simulink model "curiosity_i2c_pitch_roll"  (R2024b)
settings: Solver=FixedStepDiscrete  StartTime=0.0  StopTime=inf  FixedStep=1e-3  RelTol=1e-3  EnableMultiTasking=on
undefined symbols (not defined in the file): A0, ADC, D10, D7, D8, D9, DiscIntNeverNeededParam, Max, MaxPer, ms, NumBits1, NumBits2, P1, P58, P59, Pin, Resol, s, Timer, us
libraries: MCHP_Blockset x18, simulink x15, dspstat3 x1
(part 3 of 4)

== system curiosity_i2c_pitch_roll/Final_roll_pitch ==
  Roll_Accel : Inport
  Pitch_Accel : Inport  Port=2
  Roll_Gyro : Inport  Port=3
  Pitch_Gyro : Inport  Port=4
  Add1 : Sum
  Add2 : Sum
  HPF : Subsystem
  HPF1 : Subsystem
  LPF : Subsystem
  LPF1 : Subsystem
  Roll : Outport
  Pitch : Outport  Port=2
  wires:
  Add1/1 -> Pitch/1
  Roll_Accel/1 -> LPF/1("Rollin ")
  Roll_Gyro/1 -> HPF/1("Rollin ")
  LPF/1(Rollout) -> Add2/1
  HPF/1(Rollout) -> Add2/2
  Add2/1 -> Roll/1
  Pitch_Accel/1 -> LPF1/1(Pitchin)
  Pitch_Gyro/1 -> HPF1/1(Pitchin)
  LPF1/1(Pitchout) -> Add1/1
  HPF1/1(Pitchout) -> Add1/2

== system curiosity_i2c_pitch_roll/Gyro_bias_clculator ==
  Gx : Inport
  Gy : Inport  Port=2
  Gz : Inport  Port=3
  Enable : EnablePort
  Data Type Conversion3 : DataTypeConversion  Commented=on  OutDataTypeStr=single  SaturateOnIntegerOverflow=off  RndMeth=Floor
  Mean3 : dspstat3/Mean  Commented=on  run=on  InputProcessing=Columns as channels (frame based)  reset_popup=None  directionMode=Each column  dimension=1  roiEnable=off  roiType=Rectangles  roiPortion=Entire ROI  roiOutput=Individual statistics for each ROI  roiFlag=off  roundingMode=Floor  overflowMode=off  outputDataTypeStr=Inherit: Same as accumulator  outputMin=[]  outputMax=[]  outputLastDataTypeStr=Inherit: Same as accumulator
  manu_mean1 : Subsystem
  manu_mean2 : Subsystem
  manu_mean3 : Subsystem
  Gx_bias : Outport
  Gy_bias : Outport  Port=2
  Gz_bias : Outport  Port=3
  wires:
  Gx/1 -> manu_mean3/1(Ax)
  manu_mean3/1(Ax_bias1) -> Gx_bias/1
  Mean3/1 -> ?
  ? -> Data Type Conversion3/1
  Data Type Conversion3/1 -> Mean3/1
  manu_mean1/1(Ax_bias1) -> Gy_bias/1
  Gy/1 -> manu_mean1/1(Ax)
  Gz/1 -> manu_mean2/1(Ax)
  manu_mean2/1(Ax_bias1) -> Gz_bias/1

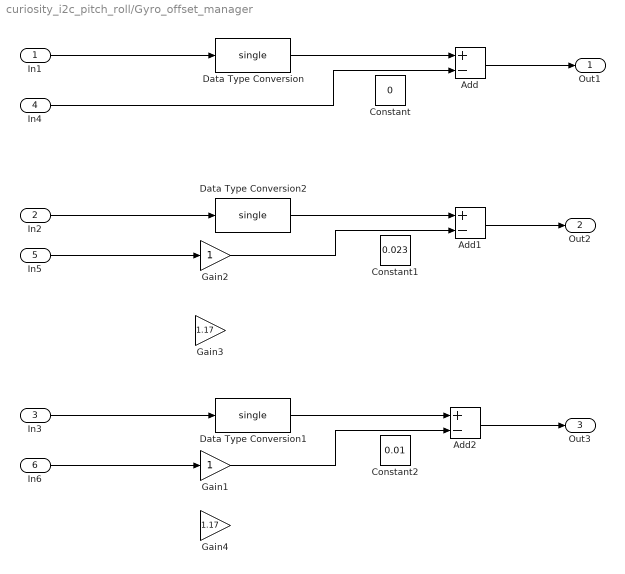
== system curiosity_i2c_pitch_roll/Gyro_offset_manager ==
  In1 : Inport
  In2 : Inport  Port=2
  In3 : Inport  Port=3
  In4 : Inport  Port=4
  In5 : Inport  Port=5
  In6 : Inport  Port=6
  Add : Sum  Inputs=+-
  Add1 : Sum  Inputs=+-
  Add2 : Sum  Inputs=+-
  Constant : Constant  Value=0  SampleTime=0.005
  Constant1 : Constant  Value=0.023  SampleTime=0.005
  Constant2 : Constant  Value=0.01  SampleTime=0.005
  Data Type Conversion : DataTypeConversion  OutDataTypeStr=single  SaturateOnIntegerOverflow=off  RndMeth=Floor
  Data Type Conversion1 : DataTypeConversion  OutDataTypeStr=single  SaturateOnIntegerOverflow=off  RndMeth=Floor
  Data Type Conversion2 : DataTypeConversion  OutDataTypeStr=single  SaturateOnIntegerOverflow=off  RndMeth=Floor
  Gain1 : Gain
  Gain2 : Gain
  Gain3 : Gain  Gain=1.17
  Gain4 : Gain  Gain=1.17
  Out1 : Outport
  Out2 : Outport  Port=2
  Out3 : Outport  Port=3
  wires:
  In3/1 -> Data Type Conversion1/1
  In1/1 -> Data Type Conversion/1
  In2/1 -> Data Type Conversion2/1
  Data Type Conversion/1 -> Add/1
  Data Type Conversion2/1 -> Add1/1
  Data Type Conversion1/1 -> Add2/1
  Add/1 -> Out1/1
  Add1/1 -> Out2/1
  Add2/1 -> Out3/1
  In5/1 -> Gain2/1
  In6/1 -> Gain1/1
  In4/1 -> Add/2
  Gain1/1 -> Add2/2
  Gain2/1 -> Add1/2

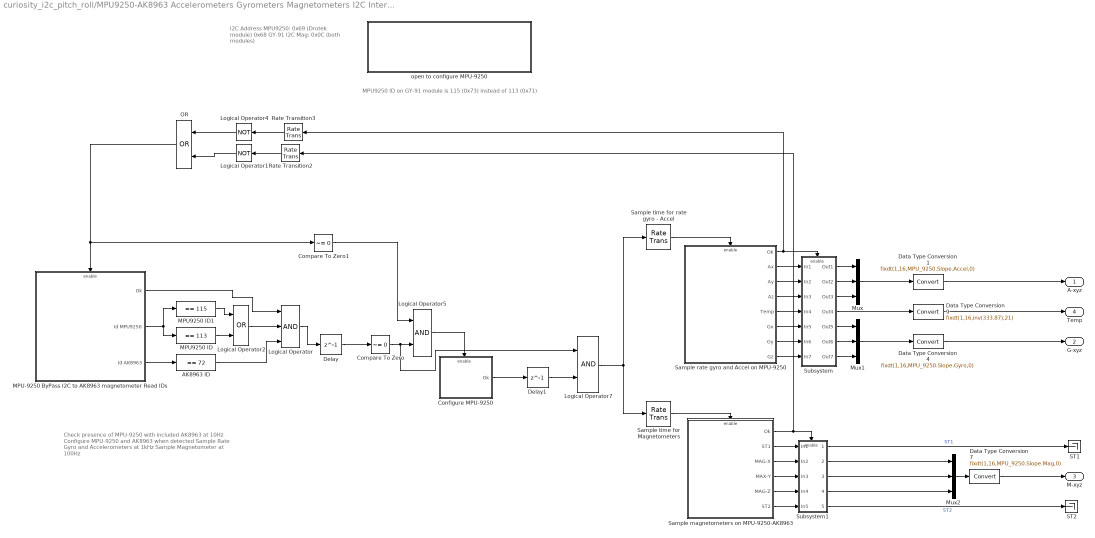
== system curiosity_i2c_pitch_roll/MPU9250-AK8963 Accelerometers Gyrometers Magnetometers I2C Interface ==
  note: I2C Address MPU9250:
      | 0x69 (Drotek module)
      | 0x68 GY-91
      |
      | I2C Mag:
      | 0x0C (both modules)
  note: MPU9250 ID on GY-91 module is 115 (0x73) instead of 113 (0x71)
  note: Check presence of MPU-9250 with included AK8963 at 10Hz
      | Configure MPU-9250 and AK8963 when detected
      | Sample Rate Gyro and Accelerometers at 1kHz
      | Sample Magnetometer at 100Hz
  AK8963 ID : simulink/Logic and Bit Operations/Compare To Constant  relop===  const=72  OutDataTypeStr=boolean
  Compare To Zero : simulink/Logic and Bit Operations/Compare To Zero  relop=~=  OutDataTypeStr=boolean
  Compare To Zero1 : simulink/Logic and Bit Operations/Compare To Zero  relop=~=  OutDataTypeStr=boolean
  Configure MPU-9250 : Subsystem  Priority=-90
  Data Type Conversion1 : DataTypeConversion  OutDataTypeStr=fixdt(1,16,MPU_9250.Slope.Accel,0)  ConvertRealWorld=Stored Integer (SI)  SaturateOnIntegerOverflow=off  RndMeth=Floor
  Data Type Conversion4 : DataTypeConversion  OutDataTypeStr=fixdt(1,16,MPU_9250.Slope.Gyro,0)  ConvertRealWorld=Stored Integer (SI)  SaturateOnIntegerOverflow=off  RndMeth=Floor
  Data Type Conversion7 : DataTypeConversion  OutDataTypeStr=fixdt(1,16,MPU_9250.Slope.Mag,0)  ConvertRealWorld=Stored Integer (SI)  SaturateOnIntegerOverflow=off  RndMeth=Floor
  Data Type Conversion9 : DataTypeConversion  OutDataTypeStr=fixdt(1,16,inv(333.87),21)  ConvertRealWorld=Stored Integer (SI)  SaturateOnIntegerOverflow=off  RndMeth=Floor
  Delay : Delay  DelayLength=1  InitialCondition=0
  Delay1 : Delay  DelayLength=1  InitialCondition=0
  Logical Operator : Logic  Inputs=3  AllPortsSameDT=off  OutDataTypeStr=boolean
  Logical Operator1 : Logic  Operator=NOT  AllPortsSameDT=off  OutDataTypeStr=boolean
  Logical Operator2 : Logic  Operator=OR  AllPortsSameDT=off  OutDataTypeStr=boolean
  Logical Operator4 : Logic  Operator=NOT  AllPortsSameDT=off  OutDataTypeStr=boolean
  Logical Operator5 : Logic  AllPortsSameDT=off  OutDataTypeStr=boolean
  Logical Operator7 : Logic  AllPortsSameDT=off  OutDataTypeStr=boolean
  MPU-9250 ByPass I2C to AK8963 magnetometer Read IDs : Subsystem
  MPU9250 ID : simulink/Logic and Bit Operations/Compare To Constant  relop===  const=113  OutDataTypeStr=boolean
  MPU9250 ID1 : simulink/Logic and Bit Operations/Compare To Constant  relop===  const=115  OutDataTypeStr=boolean
  Mux : Mux  Inputs=3
  Mux1 : Mux  Inputs=3
  Mux2 : Mux  Inputs=3
  OR : Logic  Operator=OR  AllPortsSameDT=off  OutDataTypeStr=boolean
  Rate Transition2 : RateTransition  Deterministic=off
  Rate Transition3 : RateTransition  Deterministic=off
  ST1 : Terminator
  ST2 : Terminator
  Sample magnetometers on MPU-9250-AK8963 : Subsystem
  Sample rate gyro and Accel on MPU-9250 : Subsystem  Priority=0
  Sample time for rate gyro - Accel : RateTransition  Deterministic=off  OutPortSampleTime=.005
  Sample time for Magnetometers : RateTransition  Deterministic=off  OutPortSampleTime=[.01 0.003]
  Subsystem : Subsystem
  Subsystem1 : Subsystem
  open to configure MPU-9250 : Subsystem  Priority=-500  LoadFcn=|  mask{ADDR=0x68 with AD0 Logic Low, GYRO_FS_SEL=250 deg/s, GYRO_DLPFCFG=92Hz - 3.9ms delay (Fs=1kHz), ACCEL_FS_SEL=4g, ACCEL_DLPFCFG=44.8 Hz - 4.88ms delay (Fs=1kHz), evalin_variableName=MPU_9250, evalin_ws=MPU_9250.Slope.Gyro=MCHP_Fun.Hex2num('3F21740AFA84AD89');MPU_9250.Slope.Accel=MCHP_Fun.Hex2num('3F539EB851EB851F');MPU_9250.Slope.Mag=0.15;MPU_9250.ADDR=104;MPU_9250.Config=2;MPU_9250.Gyro_Config=0;MPU_9250.Accel_Config=8;MPU_9250.Accel_Config2=3;}
      | txt = get_param(gcbh,'evalin_ws');
      | evalin('base',txt);
      mask prompts: ADDR "MPU9250 I2C 7 bit address"; GYRO_FS_SEL "Gyro Full Scale Select"; GYRO_DLPFCFG "Gyro Bandwidth"; ACCEL_FS_SEL "Accel Full Scale Select"; ACCEL_DLPFCFG "Accel Bandwidth"; evalin_variableName "evalin workSpace variable:"
      mask init:
      | MPU_9250.Slope.Gyro = sscanf(GYRO_FS_SEL,'%d')*2^-15*pi/180; % in radian/s
      | MPU_9250.Slope.Accel = sscanf(ACCEL_FS_SEL,'%d')*2^-15 * 9.81; % in m/s^2
      | MPU_9250.Slope.Mag = 0.15; % 0.15uT/LSB
      | 
      | switch ADDR
      |     case '0x68 with AD0 Logic Low'
      |         G_ADDR = hex2dec('68');
      |     case '0x69 with AD0 Logic High'
      |         G_ADDR = hex2dec('69');
      | end
      | 
      | switch GYRO_FS_SEL
      |     case '250 deg/s'
      |     	G_FS_SEL = 0;
      | 	case '500 deg/s'
      | 		G_FS_SEL = 1;
      | 	case '1000 deg/s'
      | 		G_FS_SEL = 2;
      | 	case '2000 deg/s'
      | 		G_FS_SEL = 3;
      | end
      | 
      | switch GYRO_DLPFCFG
      | 	case '8800Hz - 0.064ms delay (Fs=32kHz)'
      | 		FCHOICE = 0;
      | 		G_DLPF_CFG = 0; % don't care
      | 	case '3600Hz - 0.11ms delay (Fs=32kHz)'
      | 		FCHOICE = 1;
      | 		G_DLPF_CFG = 0; % don't care
      | 	case '3600Hz - 0.17ms delay (Fs=8kHz)'
      | 		FCHOICE = 3;
      | 		G_DLPF_CFG = 7;
      | 	case '250Hz - 0.97ms delay (Fs=8kHz)'
      | 		FCHOICE = 3;
      | 		G_DLPF_CFG = 0;
      | 	case '184Hz - 2.9ms delay (Fs=1kHz)'
      | 		FCHOICE = 3;
      | 		G_DLPF_CFG = 1;
      | 	case '92Hz - 3.9ms delay (Fs=1kHz)'
      | 		FCHOICE = 3;
      | 		G_DLPF_CFG = 2;
      | 	case '41Hz - 5.9ms delay (Fs=1kHz)'
      | 		FCHOICE = 3;
      | 		G_DLPF_CFG = 3;
      | 	case '20Hz - 9.9ms delay (Fs=1kHz)'
      | 		FCHOICE = 3;
      | 		G_DLPF_CFG = 4;
      | 	case '10Hz - 17.85ms delay (Fs=1kHz)'
      | 		FCHOICE = 3;
      | 		G_DLPF_CFG = 5;
      | 	case '5Hz - 33.48ms delay (Fs=1kHz)'
      | 		FCHOICE = 3;
      | 		G_DLPF_CFG = 6;      
      | end
      | 
      | switch ACCEL_FS_SEL
      | 	case '2g'
      | 		A_FS_SEL = 0;        
      | 	case '4g'
      | 		A_FS_SEL = 1;        
      | 	case '8g'
      | 		A_FS_SEL = 2;        
      | 	case '16g'
      | 		A_FS_SEL = 3;        
      | end
      | 
      | switch ACCEL_DLPFCFG
      | 	case '1046 Hz - 0.0503ms delay (Fs=4kHz)'
      | 		A_FCHOICE_B = 0;
      | 		A_DLPF_CFG = 0; % don't care
      | 	case '420.0 Hz - 1.38ms delay (Fs=1kHz)'
      | 		A_FCHOICE_B = 1;
      | 		A_DLPF_CFG = 7;
      | 	case '218.1 Hz - 1.88ms delay (Fs=1kHz)'
      | 		A_FCHOICE_B = 1;
      | 		A_DLPF_CFG = 1;
      | 	case '99.0 Hz - 2.88ms delay (Fs=1kHz)'
      | 		A_FCHOICE_B = 1;
      | 		A_DLPF_CFG = 2;
      | 	case '44.8 Hz - 4.88ms delay (Fs=1kHz)'
      | 		A_FCHOICE_B = 1;
      | 		A_DLPF_CFG = 3;
      | 	case '21.2 Hz - 8.87ms delay (Fs=1kHz)'
      | 		A_FCHOICE_B = 1;
      | 		A_DLPF_CFG = 4;
      | 	case '10.2 Hz - 16.83ms delay (Fs=1kHz)'
      | 		A_FCHOICE_B = 1;
      | 		A_DLPF_CFG = 5;
      | 	case '5.05 Hz - 32.48ms delay (Fs=1kHz)'
      | 		A_FCHOICE_B = 1;
      | 		A_DLPF_CFG = 6;
      | end
      | 
      | 
      | MPU_9250.ADDR = G_ADDR;
      | MPU_9250.Config = G_DLPF_CFG;
      | MPU_9250.Gyro_Config = G_FS_SEL * 2^3 + bitxor(FCHOICE,3);
      | MPU_9250.Accel_Config = A_FS_SEL * 2^3;
      | MPU_9250.Accel_Config2 = bitxor(A_FCHOICE_B,1)*2^2 + A_DLPF_CFG;
      | 
      | txt = MCHP_Fun.Struct2txt(MPU_9250,evalin_variableName);
      | set_param(gcbh,'evalin_ws',txt);
      | 
      | assignin('base',evalin_variableName,MPU_9250);
      | 
      | %mdlWks = get_param(bdroot,'ModelWorkspace');
      | %assignin(mdlWks,'MPU_9250',MPU_9250);
      mask TypeOptions ADDR: 0x68 with AD0 Logic Low | 0x69 with AD0 Logic High
      mask TypeOptions GYRO_FS_SEL: 250 deg/s | 500 deg/s | 1000 deg/s | 2000 deg/s
      mask TypeOptions GYRO_DLPFCFG: 8800Hz - 0.064ms delay (Fs=32kHz) | 3600Hz - 0.11ms delay (Fs=32kHz) | 3600Hz - 0.17ms delay (Fs=8kHz) | 250Hz - 0.97ms delay (Fs=8kHz) | 184Hz - 2.9ms delay (Fs=1kHz) | 92Hz - 3.9ms delay (Fs=1kHz) | 41Hz - 5.9ms delay (Fs=1kHz) | 20Hz - 9.9ms delay (Fs=1kHz) | 10Hz - 17.85ms delay (Fs=1kHz) | 5Hz - 33.48ms delay (Fs=1kHz)
      mask TypeOptions ACCEL_FS_SEL: 2g | 4g | 8g | 16g
      mask TypeOptions ACCEL_DLPFCFG: 1046 Hz - 0.0503ms delay (Fs=4kHz) | 420.0 Hz - 1.38ms delay (Fs=1kHz) | 218.1 Hz - 1.88ms delay (Fs=1kHz) | 99.0 Hz - 2.88ms delay (Fs=1kHz) | 44.8 Hz - 4.88ms delay (Fs=1kHz) | 21.2 Hz - 8.87ms delay (Fs=1kHz) | 10.2 Hz - 16.83ms delay (Fs=1kHz) | 5.05 Hz - 32.48ms delay (Fs=1kHz)
      mask Display: disp(['MPU-9250\n\nG: +-' GYRO_FS_SEL ' - ' GYRO_DLPFCFG '\nA: +-' ACCEL_FS_SEL ' - ' ACCEL_DLPFCFG '\nvariable --> ' evalin_variableName]);
  A-xyz : Outport  Unit=m/s^2  VectorParamsAs1DForOutWhenUnconnected=off
  G-xyz : Outport  Port=2  Unit=rad/s  VectorParamsAs1DForOutWhenUnconnected=off
  M-xyz : Outport  Port=3  Unit=µT  VectorParamsAs1DForOutWhenUnconnected=off
  Temp : Outport  Port=4  Unit=°C  VectorParamsAs1DForOutWhenUnconnected=off
  wires:
  Delay1/1 -> Logical Operator7/2
  MPU-9250 ByPass I2C to AK8963 magnetometer Read IDs/1(Ok) -> Logical Operator/1
  Logical Operator5/1 -> Configure MPU-9250/Enable
  Compare To Zero1/1 -> Logical Operator5/1
  Delay/1 -> Compare To Zero/1
  Compare To Zero/1 -> Logical Operator5/2, Logical Operator7/1
  OR/1 -> Compare To Zero1/1, MPU-9250 ByPass I2C to AK8963 magnetometer Read IDs/Enable
  Subsystem1/5(Out5) -> ST2/1  "ST2"
  Subsystem1/4(Out4) -> Mux2/3
  Subsystem1/3(Out3) -> Mux2/2
  Subsystem1/2(Out2) -> Mux2/1
  Subsystem1/1(Out1) -> ST1/1  "ST1"
  Sample magnetometers on MPU-9250-AK8963/6(ST2) -> Subsystem1/5(In5)
  Sample magnetometers on MPU-9250-AK8963/5(MAG-Z) -> Subsystem1/4(In4)
  Sample magnetometers on MPU-9250-AK8963/4(MAX-Y) -> Subsystem1/3(In3)
  Sample magnetometers on MPU-9250-AK8963/3(MAG-X) -> Subsystem1/2(In2)
  Sample magnetometers on MPU-9250-AK8963/2(ST1) -> Subsystem1/1(In1)
  Subsystem/7(Out7) -> Mux1/3
  Subsystem/6(Out6) -> Mux1/2
  Subsystem/5(Out5) -> Mux1/1
  Subsystem/4(Out4) -> Data Type Conversion9/1
  Subsystem/3(Out3) -> Mux/3
  Subsystem/2(Out2) -> Mux/2
  Subsystem/1(Out1) -> Mux/1
  Sample rate gyro and Accel on MPU-9250/8(Gz) -> Subsystem/7(In7)
  Sample rate gyro and Accel on MPU-9250/7(Gy) -> Subsystem/6(In6)
  Sample rate gyro and Accel on MPU-9250/6(Gx) -> Subsystem/5(In5)
  Sample rate gyro and Accel on MPU-9250/5(Temp) -> Subsystem/4(In4)
  Sample rate gyro and Accel on MPU-9250/4(Az) -> Subsystem/3(In3)
  Sample rate gyro and Accel on MPU-9250/3(Ay) -> Subsystem/2(In2)
  Sample rate gyro and Accel on MPU-9250/2(Ax) -> Subsystem/1(In1)
  Data Type Conversion4/1 -> G-xyz/1
  Data Type Conversion9/1 -> Temp/1
  Data Type Conversion1/1 -> A-xyz/1
  Logical Operator7/1 -> Sample time for rate gyro - Accel/1, Sample time for Magnetometers/1
  Configure MPU-9250/1(Ok) -> Delay1/1
  Logical Operator/1 -> Delay/1
  Sample time for Magnetometers/1 -> Sample magnetometers on MPU-9250-AK8963/Enable
  MPU9250 ID/1 -> Logical Operator2/2
  Sample time for rate gyro - Accel/1 -> Sample rate gyro and Accel on MPU-9250/Enable
  Logical Operator1/1 -> OR/2
  Logical Operator2/1 -> Logical Operator/2
  Mux2/1 -> Data Type Conversion7/1
  Logical Operator4/1 -> OR/1
  Rate Transition2/1 -> Logical Operator1/1
  MPU-9250 ByPass I2C to AK8963 magnetometer Read IDs/2(Id MPU9250) -> MPU9250 ID1/1, MPU9250 ID/1
  Data Type Conversion7/1 -> M-xyz/1
  MPU-9250 ByPass I2C to AK8963 magnetometer Read IDs/3("Id AK8963 ") -> AK8963 ID/1
  Mux/1 -> Data Type Conversion1/1
  Sample magnetometers on MPU-9250-AK8963/1(Ok) -> Rate Transition2/1, Subsystem1/Enable
  AK8963 ID/1 -> Logical Operator/3
  MPU9250 ID1/1 -> Logical Operator2/1
  Rate Transition3/1 -> Logical Operator4/1
  Sample rate gyro and Accel on MPU-9250/1(Ok) -> Subsystem/Enable, Rate Transition3/1
  Mux1/1 -> Data Type Conversion4/1

== system curiosity_i2c_pitch_roll/Roll_&_Pitch_Acel ==
  Ax : Inport
  Ay : Inport  Port=2
  Az : Inport  Port=3
  Add : Sum
  Ay1 : InportShadow  Port=2
  Az1 : InportShadow  Port=3
  Gain : Gain  Gain=-1
  Gain1 : Gain  Gain=57.29
  Gain2 : Gain  Gain=57.29
  Sqrt : Sqrt
  Square : Math  Operator=square
  Square1 : Math  Operator=square
  Trigonometric Function1 : Trigonometry  Operator=atan2  ApproximationMethod=Lookup  TableDataTypeStr=single
  Trigonometric Function2 : Trigonometry  Operator=atan2  ApproximationMethod=Lookup  TableDataTypeStr=single
  Roll_angle : Outport
  Pitch_angle : Outport  Port=2
  wires:
  Square1/1 -> Add/2
  Gain/1 -> Trigonometric Function2/1
  Sqrt/1 -> Trigonometric Function2/2
  Add/1 -> Sqrt/1
  Square/1 -> Add/1
  Ay/1 -> Trigonometric Function1/1
  Az/1 -> Trigonometric Function1/2
  Trigonometric Function1/1 -> Gain1/1
  Ax/1 -> Gain/1
  Ay1/1 -> Square/1
  Az1/1 -> Square1/1
  Trigonometric Function2/1 -> Gain2/1
  Gain1/1 -> Roll_angle/1
  Gain2/1 -> Pitch_angle/1

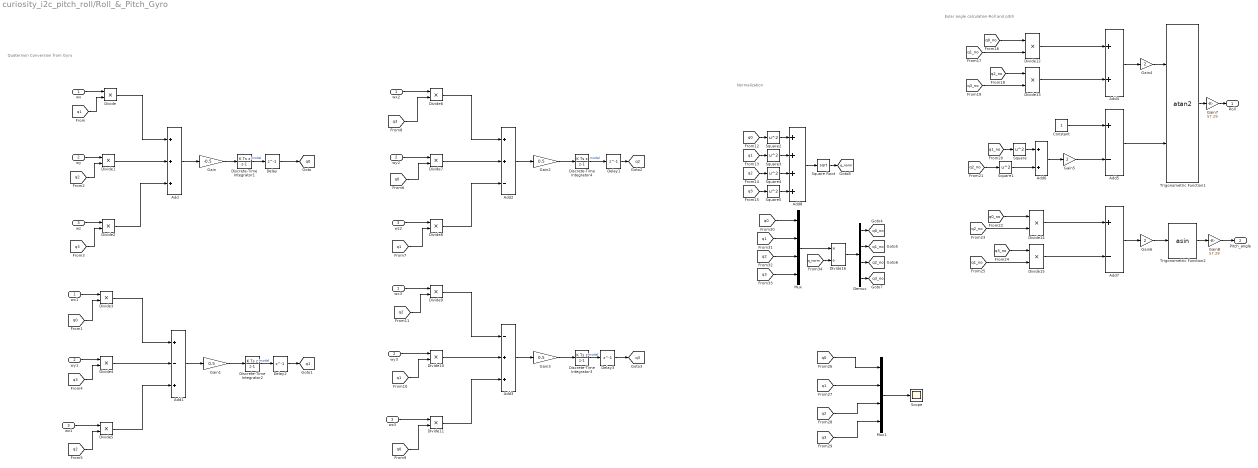
== system curiosity_i2c_pitch_roll/Roll_&_Pitch_Gyro ==
  note: Eular angle calculation-Roll and pitch
  note: Normalization
  note: Quaternion Conversion from Gyro
  wx : Inport
  wy : Inport  Port=2
  wz : Inport  Port=3
  Add : Sum  Inputs=+++
  Add1 : Sum  Inputs=+-+
  Add2 : Sum  Inputs=++-
  Add3 : Sum  Inputs=-++
  Add4 : Sum
  Add5 : Sum  Inputs=+-
  Add6 : Sum
  Add7 : Sum  Inputs=+-
  Add8 : Sum  Inputs=++++
  Constant : Constant  OutDataTypeStr=single  SampleTime=0.005
  Delay : Delay  DelayLength=1  InitialCondition=1  InputProcessing=Columns as channels (frame based)
  Delay1 : Delay  DelayLength=1  InputProcessing=Columns as channels (frame based)
  Delay2 : Delay  DelayLength=1  InputProcessing=Columns as channels (frame based)
  Delay3 : Delay  DelayLength=1  InputProcessing=Columns as channels (frame based)
  Demux : Demux
  Discrete-Time Integrator1 : DiscreteIntegrator  IntegratorMethod=Integration: Backward Euler  InitialCondition=1  SampleTime=-1  OutDataTypeStr=single  ICPrevOutput=DiscIntNeverNeededParam  ICPrevScaledInput=DiscIntNeverNeededParam
  Discrete-Time Integrator2 : DiscreteIntegrator  IntegratorMethod=Integration: Backward Euler  SampleTime=-1  OutDataTypeStr=single  ICPrevOutput=DiscIntNeverNeededParam  ICPrevScaledInput=DiscIntNeverNeededParam
  Discrete-Time Integrator3 : DiscreteIntegrator  IntegratorMethod=Integration: Backward Euler  SampleTime=-1  OutDataTypeStr=single  ICPrevOutput=DiscIntNeverNeededParam  ICPrevScaledInput=DiscIntNeverNeededParam
  Discrete-Time Integrator4 : DiscreteIntegrator  IntegratorMethod=Integration: Backward Euler  SampleTime=-1  OutDataTypeStr=single  ICPrevOutput=DiscIntNeverNeededParam  ICPrevScaledInput=DiscIntNeverNeededParam
  Divide{,1..15} (16 alike) : Product  Inputs=**
  Divide16 : Product  Inputs=*/
  Gain : Gain  Gain=-0.5
  Gain1 : Gain  Gain=0.5
  Gain2 : Gain  Gain=0.5
  Gain3 : Gain  Gain=0.5
  Gain4 : Gain  Gain=2
  Gain5 : Gain  Gain=2
  Gain6 : Gain  Gain=2
  Gain7 : Gain  Gain=57.29
  Gain8 : Gain  Gain=57.29
  Mux : Mux
  Mux1 : Mux
  Scope : Scope
  Square{,1..5} (6 alike) : Math  Operator=square
  Square Root : Sqrt
  Trigonometric Function1 : Trigonometry  Operator=atan2  ApproximationMethod=Lookup  TableDataTypeStr=single
  Trigonometric Function2 : Trigonometry  Operator=asin  ApproximationMethod=Lookup  TableDataTypeStr=single
  wx1 : InportShadow
  wx2 : InportShadow
  wx3 : InportShadow
  wy1 : InportShadow  Port=2
  wy2 : InportShadow  Port=2
  wy3 : InportShadow  Port=2
  wz1 : InportShadow  Port=3
  wz2 : InportShadow  Port=3
  wz3 : InportShadow  Port=3
  Roll : Outport
  Pitch_angle : Outport  Port=2
  tag scope: q0=global, q0_no=global, q1=global, q1_no=global, q2=global, q2_no=global, q3=global, q3_no=global, q_norm=global
  wires:
  [q0] -> Square2/1
  [q1] -> Square3/1
  [q2] -> Square4/1
  [q3] -> Square5/1
  Divide12/1 -> Add4/1
  [q1_no] -> Divide12/2
  [q2_no] -> Divide13/1
  Divide13/1 -> Add4/2
  [q3_no] -> Divide13/2
  Add4/1 -> Gain4/1
  Gain4/1 -> Trigonometric Function1/1
  Constant/1 -> Add5/1
  Gain5/1 -> Add5/2
  [q1_no] -> Square/1
  Add6/1 -> Gain5/1
  Square/1 -> Add6/1
  [q2_no] -> Square1/1
  Square1/1 -> Add6/2
  Add5/1 -> Trigonometric Function1/2
  [q1_no] -> Divide15/2
  Divide15/1 -> Add7/2
  [q3_no] -> Divide15/1
  [q2_no] -> Divide14/2
  [q0_no] -> Divide14/1
  Divide14/1 -> Add7/1
  Add7/1 -> Gain6/1
  Gain6/1 -> Trigonometric Function2/1
  Trigonometric Function2/1 -> Gain8/1
  [q0] -> Mux1/1
  Mux1/1 -> Scope/1
  [q1] -> Mux1/2
  [q2] -> Mux1/3
  [q3] -> Mux1/4
  Square2/1 -> Add8/1
  Square3/1 -> Add8/2
  Square4/1 -> Add8/3
  Square5/1 -> Add8/4
  Add8/1 -> Square Root/1
  Square Root/1 -> [q_norm]
  [q0] -> Mux/1
  [q1] -> Mux/2
  [q2] -> Mux/3
  [q3] -> Mux/4
  Mux/1 -> Divide16/1
  [q_norm] -> Divide16/2
  Divide16/1 -> Demux/1
  Demux/1 -> [q0_no]
  Demux/2 -> [q1_no]
  Demux/3 -> [q2_no]
  Demux/4 -> [q3_no]
  [q0_no] -> Divide12/1
  Divide4/1 -> Add1/2
  Add3/1 -> Gain3/1
  Add1/1 -> Gain1/1
  Divide9/1 -> Add3/1
  Discrete-Time Integrator1/1 -> Delay/1  "model"
  Divide11/1 -> Add3/3
  wz1/1 -> Divide5/1
  Delay2/1 -> [q1]
  wx/1 -> Divide/1
  Discrete-Time Integrator2/1 -> Delay2/1  "model"
  Divide8/1 -> Add2/3
  wx2/1 -> Divide6/1
  [q0] -> Divide11/2
  Gain/1 -> Discrete-Time Integrator1/1
  wx1/1 -> Divide3/1
  Divide/1 -> Add/1
  [q3] -> Divide4/2
  wz2/1 -> Divide8/1
  Discrete-Time Integrator3/1 -> Delay3/1  "model"
  wx3/1 -> Divide9/1
  Divide3/1 -> Add1/1
  [q3] -> Divide2/2
  Add2/1 -> Gain2/1
  Add/1 -> Gain/1
  Divide2/1 -> Add/3
  Discrete-Time Integrator4/1 -> Delay1/1  "model"
  [q2] -> Divide5/2
  Delay1/1 -> [q2]
  wz/1 -> Divide2/1
  wy/1 -> Divide1/1
  [q2] -> Divide9/2
  Divide7/1 -> Add2/2
  [q2] -> Divide1/2
  Gain2/1 -> Discrete-Time Integrator4/1
  [q0] -> Divide7/2
  Divide5/1 -> Add1/3
  wy3/1 -> Divide10/1
  Divide1/1 -> Add/2
  Gain3/1 -> Discrete-Time Integrator3/1
  Gain1/1 -> Discrete-Time Integrator2/1
  Divide10/1 -> Add3/2
  Divide6/1 -> Add2/1
  [q3] -> Divide6/2
  wy1/1 -> Divide4/1
  Delay/1 -> [q0]
  wy2/1 -> Divide7/1
  Delay3/1 -> [q3]
  [q1] -> Divide10/2
  [q1] -> Divide8/2
  [q0] -> Divide3/2
  wz3/1 -> Divide11/1
  [q1] -> Divide/2
  Trigonometric Function1/1 -> Gain7/1
  Gain7/1 -> Roll/1
  Gain8/1 -> Pitch_angle/1

== system curiosity_i2c_pitch_roll/Sine Wave Generator Use dsPIC A hardware sine fct ==
  In1 : Inport
  Bias : Bias  Bias=0.5  SaturateOnIntegerOverflow=off
  Cast3 : DataTypeConversion  OutDataTypeStr=single  SaturateOnIntegerOverflow=off  RndMeth=Floor
  Discrete-Time Integrator3 : DiscreteIntegrator  gainval=1  SampleTime=.01  OutDataTypeStr=fixdt(0,16,16)  RndMeth=Simplest  ICPrevOutput=DiscIntNeverNeededParam  ICPrevScaledInput=DiscIntNeverNeededParam
      settings: LockScale=on
  Gain : Gain  Gain=0.5
  Gain2 : Gain  Gain=2*pi
  Sin3 : Trigonometry  OutputSignalType=real
  Out1 : Outport
  wires:
  In1/1 -> Discrete-Time Integrator3/1
  Discrete-Time Integrator3/1 -> Cast3/1
  Bias/1 -> Out1/1
  Gain2/1 -> Sin3/1
  Sin3/1 -> Gain/1
  Cast3/1 -> Gain2/1
  Gain/1 -> Bias/1

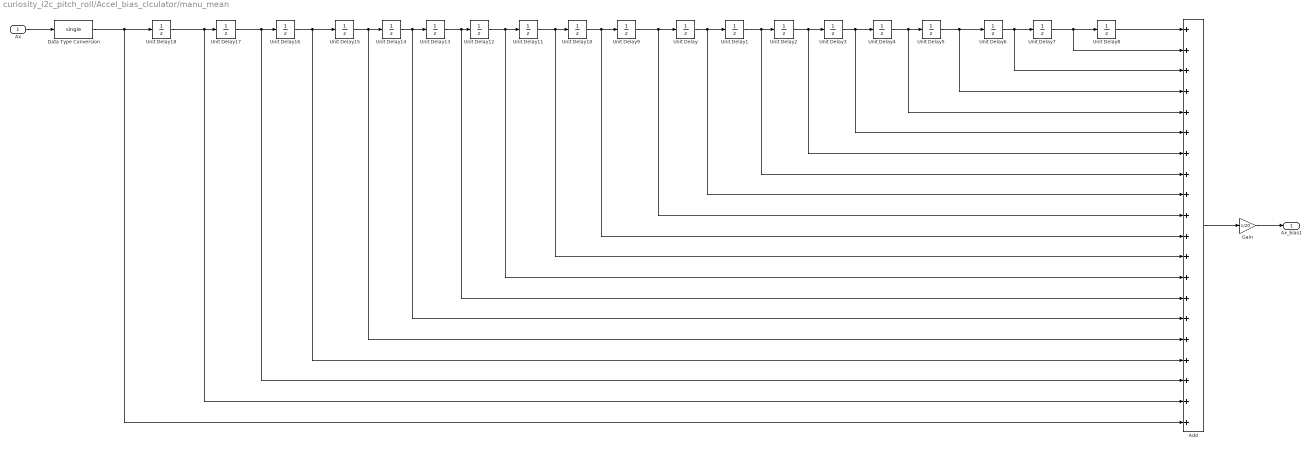
== system curiosity_i2c_pitch_roll/Accel_bias_clculator/manu_mean ==
  Ax : Inport
  Add : Sum  Inputs=++++++++++++++++++++
  Data Type Conversion : DataTypeConversion  OutDataTypeStr=single  SaturateOnIntegerOverflow=off  RndMeth=Floor
  Gain : Gain  Gain=1/20
  Unit Delay{,1..18} (19 alike) : UnitDelay  SampleTime=-1  HasFrameUpgradeWarning=on
  Ax_bias1 : Outport
  wires:
  Unit Delay2/1 -> Add/7, Unit Delay3/1
  Unit Delay1/1 -> Add/8, Unit Delay2/1
  Unit Delay/1 -> Add/9, Unit Delay1/1
  Unit Delay7/1 -> Add/2, Unit Delay8/1
  Unit Delay5/1 -> Add/4, Unit Delay6/1
  Unit Delay4/1 -> Add/5, Unit Delay5/1
  Unit Delay3/1 -> Add/6, Unit Delay4/1
  Unit Delay6/1 -> Add/3, Unit Delay7/1
  Data Type Conversion/1 -> Add/20, Unit Delay18/1
  Add/1 -> Gain/1
  Ax/1 -> Data Type Conversion/1
  Unit Delay8/1 -> Add/1
  Gain/1 -> Ax_bias1/1
  Unit Delay9/1 -> Add/10, Unit Delay/1
  Unit Delay10/1 -> Add/11, Unit Delay9/1
  Unit Delay11/1 -> Add/12, Unit Delay10/1
  Unit Delay12/1 -> Add/13, Unit Delay11/1
  Unit Delay13/1 -> Add/14, Unit Delay12/1
  Unit Delay14/1 -> Add/15, Unit Delay13/1
  Unit Delay15/1 -> Add/16, Unit Delay14/1
  Unit Delay16/1 -> Add/17, Unit Delay15/1
  Unit Delay17/1 -> Add/18, Unit Delay16/1
  Unit Delay18/1 -> Add/19, Unit Delay17/1

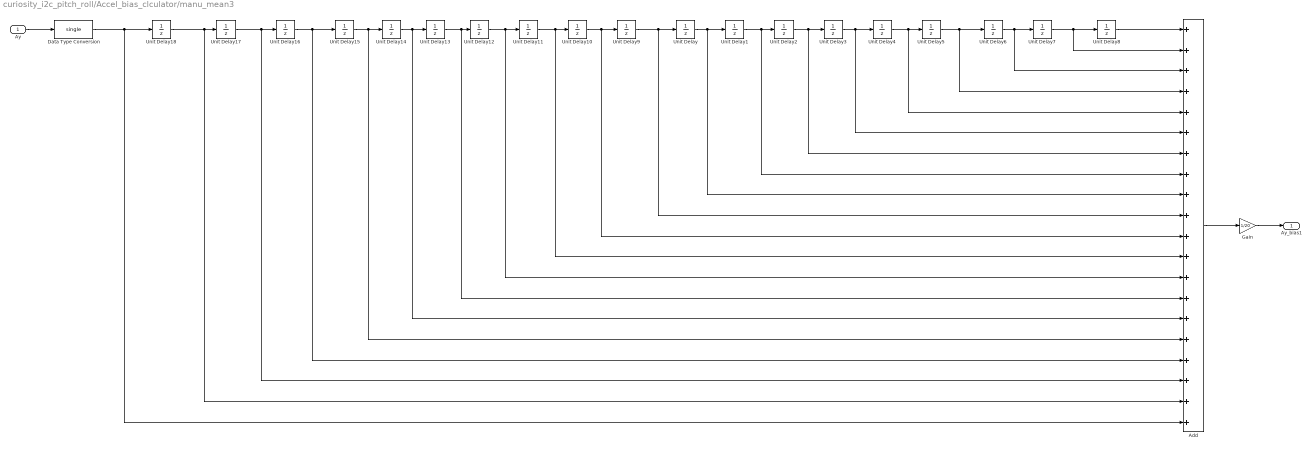
== system curiosity_i2c_pitch_roll/Accel_bias_clculator/manu_mean3 ==
  Ay : Inport
  Add : Sum  Inputs=++++++++++++++++++++
  Data Type Conversion : DataTypeConversion  OutDataTypeStr=single  SaturateOnIntegerOverflow=off  RndMeth=Floor
  Gain : Gain  Gain=1/20
  Unit Delay{,1..18} (19 alike) : UnitDelay  SampleTime=-1  HasFrameUpgradeWarning=on
  Ay_bias1 : Outport
  wires:
  Unit Delay18/1 -> Unit Delay17/1, Add/19
  Unit Delay17/1 -> Unit Delay16/1, Add/18
  Unit Delay16/1 -> Unit Delay15/1, Add/17
  Unit Delay15/1 -> Unit Delay14/1, Add/16
  Unit Delay14/1 -> Unit Delay13/1, Add/15
  Unit Delay13/1 -> Unit Delay12/1, Add/14
  Unit Delay12/1 -> Unit Delay11/1, Add/13
  Unit Delay11/1 -> Unit Delay10/1, Add/12
  Unit Delay10/1 -> Unit Delay9/1, Add/11
  Unit Delay9/1 -> Unit Delay/1, Add/10
  Gain/1 -> Ay_bias1/1
  Unit Delay8/1 -> Add/1
  Ay/1 -> Data Type Conversion/1
  Add/1 -> Gain/1
  Data Type Conversion/1 -> Unit Delay18/1, Add/20
  Unit Delay6/1 -> Unit Delay7/1, Add/3
  Unit Delay3/1 -> Unit Delay4/1, Add/6
  Unit Delay4/1 -> Unit Delay5/1, Add/5
  Unit Delay5/1 -> Unit Delay6/1, Add/4
  Unit Delay7/1 -> Unit Delay8/1, Add/2
  Unit Delay/1 -> Unit Delay1/1, Add/9
  Unit Delay1/1 -> Unit Delay2/1, Add/8
  Unit Delay2/1 -> Unit Delay3/1, Add/7

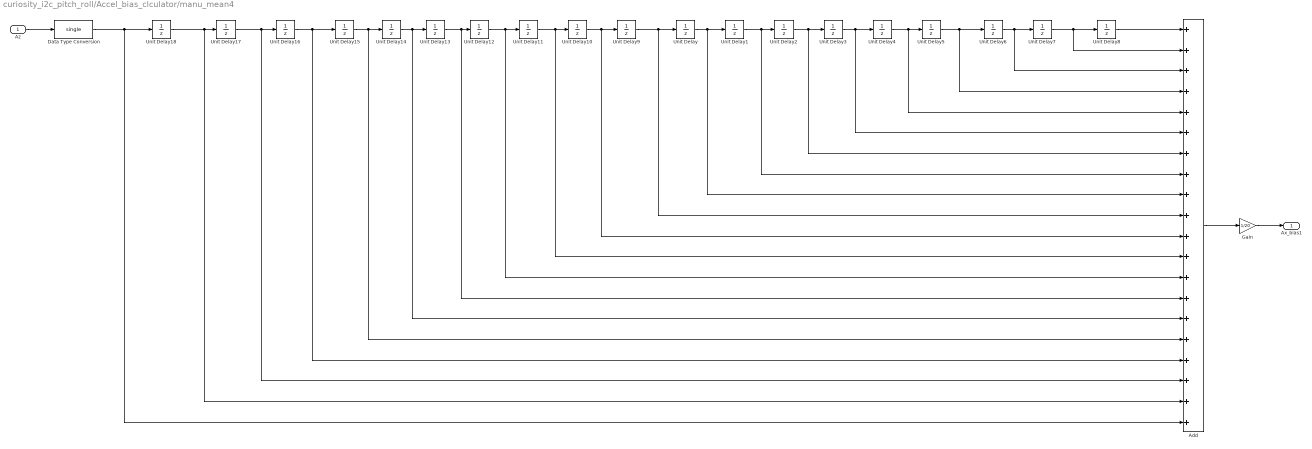
== system curiosity_i2c_pitch_roll/Accel_bias_clculator/manu_mean4 ==
  Az : Inport
  Add : Sum  Inputs=++++++++++++++++++++
  Data Type Conversion : DataTypeConversion  OutDataTypeStr=single  SaturateOnIntegerOverflow=off  RndMeth=Floor
  Gain : Gain  Gain=1/20
  Unit Delay{,1..18} (19 alike) : UnitDelay  SampleTime=-1  HasFrameUpgradeWarning=on
  Ax_bias1 : Outport
  wires:
  Unit Delay2/1 -> Add/7, Unit Delay3/1
  Unit Delay1/1 -> Add/8, Unit Delay2/1
  Unit Delay/1 -> Add/9, Unit Delay1/1
  Unit Delay7/1 -> Add/2, Unit Delay8/1
  Unit Delay5/1 -> Add/4, Unit Delay6/1
  Unit Delay4/1 -> Add/5, Unit Delay5/1
  Unit Delay3/1 -> Add/6, Unit Delay4/1
  Unit Delay6/1 -> Add/3, Unit Delay7/1
  Data Type Conversion/1 -> Add/20, Unit Delay18/1
  Add/1 -> Gain/1
  Az/1 -> Data Type Conversion/1
  Unit Delay8/1 -> Add/1
  Gain/1 -> Ax_bias1/1
  Unit Delay9/1 -> Add/10, Unit Delay/1
  Unit Delay10/1 -> Add/11, Unit Delay9/1
  Unit Delay11/1 -> Add/12, Unit Delay10/1
  Unit Delay12/1 -> Add/13, Unit Delay11/1
  Unit Delay13/1 -> Add/14, Unit Delay12/1
  Unit Delay14/1 -> Add/15, Unit Delay13/1
  Unit Delay15/1 -> Add/16, Unit Delay14/1
  Unit Delay16/1 -> Add/17, Unit Delay15/1
  Unit Delay17/1 -> Add/18, Unit Delay16/1
  Unit Delay18/1 -> Add/19, Unit Delay17/1

== system curiosity_i2c_pitch_roll/Buttosn * Pot/Downsample x10 ==
  note: DownSample & Average by changing data scaling
  In1 : Inport
  Compare To Constant : simulink/Logic and Bit Operations/Compare To Constant  relop===  const=1  OutDataTypeStr=boolean
  Counter Limited : simulink/Sources/Counter Limited  uplimit=DownSample-1  tsamp=-1
  Data Type Duplicate : DataTypeDuplicate
  Data Type Propagation : simulink/Signal Attributes/Data Type Propagation  PropDataType=fixdt(1, 16)  IfRefDouble=double  IfRefSingle=single  IsSigned=IsSigned1 or IsSigned2  NumBitsBase=NumBits1+NumBits2  NumBitsMult=1  NumBitsAdd=0  NumBitsAllowFinal=-1  PropScaling=2^-10  ValuesUsedBestPrec=[5 -7]  SlopeBase=Slope1  SlopeMult=1  SlopeAdd=0  BiasBase=Bias1  BiasMult=1  BiasAdd=0
  Data Type Propagation1 : simulink/Signal Attributes/Data Type Propagation  PropDataType=fixdt(1, 16)  IfRefDouble=double  IfRefSingle=single  IsSigned=IsSigned1 or IsSigned2  NumBitsBase=NumBits1+NumBits2  NumBitsMult=1  NumBitsAdd=0  NumBitsAllowFinal=-1  PropScaling=2^-10  ValuesUsedBestPrec=[5 -7]  SlopeBase=PosRange1  SlopeMult=1  SlopeAdd=0  BiasBase=Bias1  BiasMult=1  BiasAdd=0
  Discrete-Time Integrator : DiscreteIntegrator  IntegratorMethod=Accumulation: Backward Euler  gainval=1  ExternalReset=sampled level  SampleTime=-1  OutDataTypeStr=Inherit: Inherit via back propagation  ICPrevOutput=DiscIntNeverNeededParam  ICPrevScaledInput=DiscIntNeverNeededParam
  Gain : Gain  Gain=1/DownSample  OutDataTypeStr=Inherit: Inherit via back propagation  RndMeth=Round
  Gain1 : Gain  Gain=1/DownSample  OutDataTypeStr=Inherit: Inherit via back propagation
  Rate Transition1 : RateTransition  OutPortSampleTimeOpt=Multiple of input port sample time  OutPortSampleTimeMultiple=DownSample  OutPortSampleTime=DownSample
  Rate Transition3 : RateTransition  OutPortSampleTimeOpt=Multiple of input port sample time  OutPortSampleTimeMultiple=DownSample  OutPortSampleTime=DownSample
  Terminator : Terminator
  Out1 : Outport  VectorParamsAs1DForOutWhenUnconnected=off
  wires:
  Gain1/1 -> Data Type Propagation1/3, Terminator/1
  Rate Transition1/1 -> Data Type Duplicate/1, Data Type Propagation1/1, Data Type Propagation1/2
  Gain/1 -> Out1/1, Data Type Duplicate/2
  Counter Limited/1 -> Compare To Constant/1
  Discrete-Time Integrator/1 -> Rate Transition3/1, Data Type Propagation/3
  Compare To Constant/1 -> Discrete-Time Integrator/2
  In1/1 -> Data Type Propagation/1, Data Type Propagation/2, Discrete-Time Integrator/1, Rate Transition1/1
  Rate Transition3/1 -> Gain/1, Gain1/1

== system curiosity_i2c_pitch_roll/CuriosityPlatform Development Board dsPIC33AK128MC106 GP DIM/Timing Analysis ==
  note: CPU overload is 0 if no overload took place between two MCU Overload block execution.
      | Otherwise, bits field output code for TID(s) responsible for at least one overload.
  Downsample Averaged2 : Subsystem  mask{InputSampleTime=.001, DownSample=100}
      mask prompts: InputSampleTime "Input sample time"; DownSample "DownSample Factor"
  Gain : Gain  Gain=20e-9/.001 * 100  OutMin=0  OutMax=100  OutDataTypeStr=fixdt(0,16)  RndMeth=Simplest  SaturateOnIntegerOverflow=on
  MCU Load : MCHP_Blockset/Profiling/MCU Load  MCULoadPin_TXT=None  MCULoadMeasure=on  TIMER_Resolution_TXT="Resol: 0.02(us)  -  Max: 1.31(ms)"  MCHP_TIMER_REQUEST={MCU_Load}{MCU_Load}21:5:0:0:[]:131072;  MCHP_TIMER_RESULT=[3 65535 ]  MCHP_MASTERLINK=curiosity_i2c_pitch_roll/CuriosityPlatform Development Board dsPIC33AK128MC106 GP DIM/Microchip Master  MCHP_COMPILED_INFO="CompiledSampleTime= [0.0010000000000000000208   0 ];CompiledInportDataTypes=[    ];CompiledInportDataWidth=[];"  Info="Timer 3:  Resol: 20(ns)  -  Max: 1.31072(ms)"  SampleTime=.001
      settings: SourceProductName=MPLAB Device Blocks for Simulink
  MCU Overload : MCHP_Blockset/Profiling/MCU Overload  MCUOverloadBlockOutput=on  MCUOverLoadPin_TXT=None  MCHP_MASTERLINK=curiosity_i2c_pitch_roll/CuriosityPlatform Development Board dsPIC33AK128MC106 GP DIM/Microchip Master  SampleTime=-1
      settings: SourceProductName=MPLAB Device Blocks for Simulink
  Overload : Constant  Value=65535  OutDataTypeStr=Inherit: Inherit via back propagation
  Rate Transition : RateTransition  Deterministic=off  OutPortSampleTime=.0005*200
  Switch : Switch  Criteria=u2 ~= 0  SaturateOnIntegerOverflow=off  InputSameDT=off
  CPU Load : Outport  Unit=%  SampleTime=.0005*200
  CPU Overload : Outport  Port=2
  wires:
  Gain/1 -> CPU Load/1
  Overload/1 -> Switch/1
  Switch/1 -> Gain/1
  Downsample Averaged2/1(Out1) -> Switch/3
  MCU Load/1 -> Downsample Averaged2/1(In1)
  MCU Overload/1 -> CPU Overload/1, Rate Transition/1
  Rate Transition/1 -> Switch/2

== system curiosity_i2c_pitch_roll/Final_roll_pitch/HPF ==
  "Rollin " : Inport
  Add : Sum
  Add1 : Sum  Inputs=+-
  Gain : Gain  Gain=0.9844
  Gain1 : Gain  Gain=0.9844
  Unit Delay : UnitDelay  SampleTime=-1  HasFrameUpgradeWarning=on
  Unit Delay1 : UnitDelay  SampleTime=-1  HasFrameUpgradeWarning=on
  Rollout : Outport
  wires:
  Gain/1 -> Add/2
  Unit Delay/1 -> Gain/1
  Add/1 -> Rollout/1, Unit Delay/1
  "Rollin "/1 -> Add1/1, Unit Delay1/1
  Add1/1 -> Gain1/1
  Unit Delay1/1 -> Add1/2
  Gain1/1 -> Add/1

== system curiosity_i2c_pitch_roll/Final_roll_pitch/HPF1 ==
  Pitchin : Inport
  Add : Sum
  Add1 : Sum  Inputs=+-
  Gain : Gain  Gain=0.9844
  Gain1 : Gain  Gain=0.9844
  Unit Delay : UnitDelay  SampleTime=-1  HasFrameUpgradeWarning=on
  Unit Delay1 : UnitDelay  SampleTime=-1  HasFrameUpgradeWarning=on
  Pitchout : Outport
  wires:
  Gain/1 -> Add/2
  Unit Delay/1 -> Gain/1
  Add/1 -> Pitchout/1, Unit Delay/1
  Pitchin/1 -> Add1/1, Unit Delay1/1
  Add1/1 -> Gain1/1
  Unit Delay1/1 -> Add1/2
  Gain1/1 -> Add/1

== system curiosity_i2c_pitch_roll/Final_roll_pitch/LPF ==
  "Rollin " : Inport
  Add : Sum
  Gain : Gain  Gain=0.9844
  Gain1 : Gain  Gain=1-0.9844
  Unit Delay : UnitDelay  SampleTime=-1  HasFrameUpgradeWarning=on
  Rollout : Outport
  wires:
  Add/1 -> Unit Delay/1, Rollout/1
  Unit Delay/1 -> Gain/1
  Gain/1 -> Add/2
  Gain1/1 -> Add/1
  "Rollin "/1 -> Gain1/1

== system curiosity_i2c_pitch_roll/Final_roll_pitch/LPF1 ==
  Pitchin : Inport
  Add : Sum
  Gain : Gain  Gain=0.9844
  Gain1 : Gain  Gain=1-0.9844
  Unit Delay : UnitDelay  SampleTime=-1  HasFrameUpgradeWarning=on
  Pitchout : Outport
  wires:
  Add/1 -> Unit Delay/1, Pitchout/1
  Unit Delay/1 -> Gain/1
  Gain/1 -> Add/2
  Gain1/1 -> Add/1
  Pitchin/1 -> Gain1/1

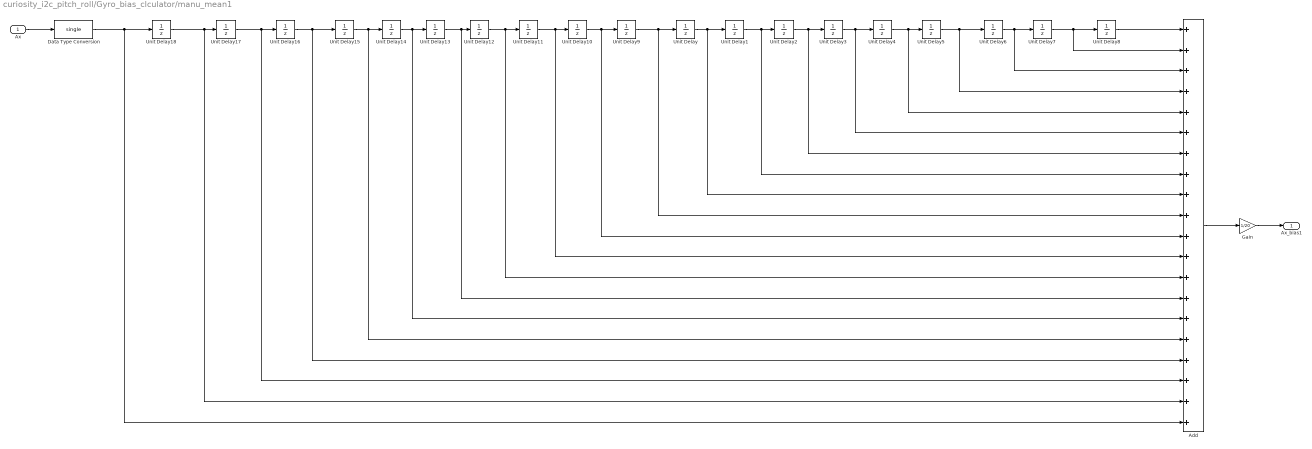
== system curiosity_i2c_pitch_roll/Gyro_bias_clculator/manu_mean1 ==
  Ax : Inport
  Add : Sum  Inputs=++++++++++++++++++++
  Data Type Conversion : DataTypeConversion  OutDataTypeStr=single  SaturateOnIntegerOverflow=off  RndMeth=Floor
  Gain : Gain  Gain=1/20
  Unit Delay{,1..18} (19 alike) : UnitDelay  SampleTime=-1  HasFrameUpgradeWarning=on
  Ax_bias1 : Outport
  wires:
  Unit Delay18/1 -> Unit Delay17/1, Add/19
  Unit Delay17/1 -> Unit Delay16/1, Add/18
  Unit Delay16/1 -> Unit Delay15/1, Add/17
  Unit Delay15/1 -> Unit Delay14/1, Add/16
  Unit Delay14/1 -> Unit Delay13/1, Add/15
  Unit Delay13/1 -> Unit Delay12/1, Add/14
  Unit Delay12/1 -> Unit Delay11/1, Add/13
  Unit Delay11/1 -> Unit Delay10/1, Add/12
  Unit Delay10/1 -> Unit Delay9/1, Add/11
  Unit Delay9/1 -> Unit Delay/1, Add/10
  Gain/1 -> Ax_bias1/1
  Unit Delay8/1 -> Add/1
  Ax/1 -> Data Type Conversion/1
  Add/1 -> Gain/1
  Data Type Conversion/1 -> Unit Delay18/1, Add/20
  Unit Delay6/1 -> Unit Delay7/1, Add/3
  Unit Delay3/1 -> Unit Delay4/1, Add/6
  Unit Delay4/1 -> Unit Delay5/1, Add/5
  Unit Delay5/1 -> Unit Delay6/1, Add/4
  Unit Delay7/1 -> Unit Delay8/1, Add/2
  Unit Delay/1 -> Unit Delay1/1, Add/9
  Unit Delay1/1 -> Unit Delay2/1, Add/8
  Unit Delay2/1 -> Unit Delay3/1, Add/7

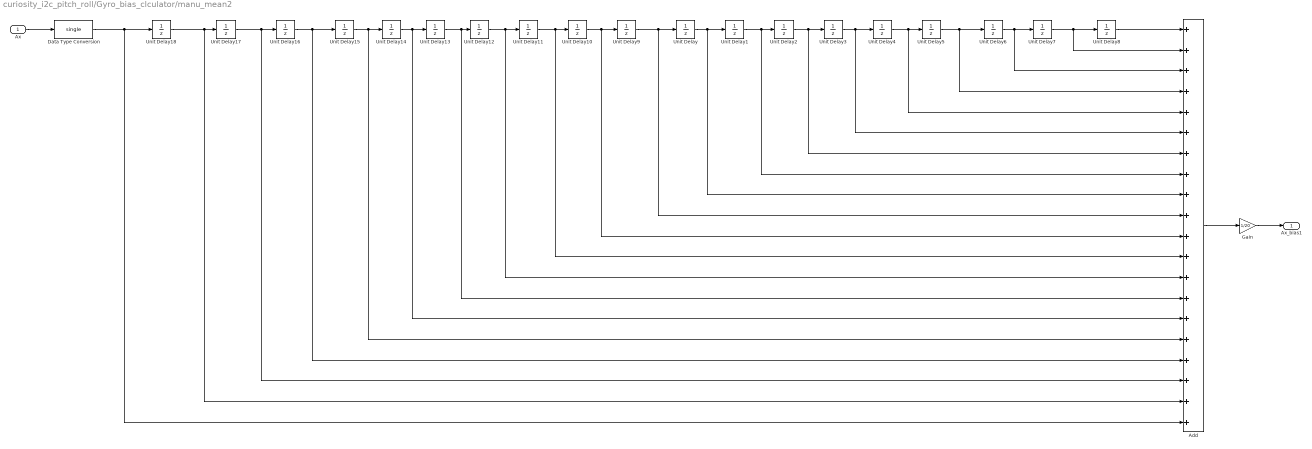
== system curiosity_i2c_pitch_roll/Gyro_bias_clculator/manu_mean2 ==
  Ax : Inport
  Add : Sum  Inputs=++++++++++++++++++++
  Data Type Conversion : DataTypeConversion  OutDataTypeStr=single  SaturateOnIntegerOverflow=off  RndMeth=Floor
  Gain : Gain  Gain=1/20
  Unit Delay{,1..18} (19 alike) : UnitDelay  SampleTime=-1  HasFrameUpgradeWarning=on
  Ax_bias1 : Outport
  wires:
  Unit Delay2/1 -> Add/7, Unit Delay3/1
  Unit Delay1/1 -> Add/8, Unit Delay2/1
  Unit Delay/1 -> Add/9, Unit Delay1/1
  Unit Delay7/1 -> Add/2, Unit Delay8/1
  Unit Delay5/1 -> Add/4, Unit Delay6/1
  Unit Delay4/1 -> Add/5, Unit Delay5/1
  Unit Delay3/1 -> Add/6, Unit Delay4/1
  Unit Delay6/1 -> Add/3, Unit Delay7/1
  Data Type Conversion/1 -> Add/20, Unit Delay18/1
  Add/1 -> Gain/1
  Ax/1 -> Data Type Conversion/1
  Unit Delay8/1 -> Add/1
  Gain/1 -> Ax_bias1/1
  Unit Delay9/1 -> Add/10, Unit Delay/1
  Unit Delay10/1 -> Add/11, Unit Delay9/1
  Unit Delay11/1 -> Add/12, Unit Delay10/1
  Unit Delay12/1 -> Add/13, Unit Delay11/1
  Unit Delay13/1 -> Add/14, Unit Delay12/1
  Unit Delay14/1 -> Add/15, Unit Delay13/1
  Unit Delay15/1 -> Add/16, Unit Delay14/1
  Unit Delay16/1 -> Add/17, Unit Delay15/1
  Unit Delay17/1 -> Add/18, Unit Delay16/1
  Unit Delay18/1 -> Add/19, Unit Delay17/1

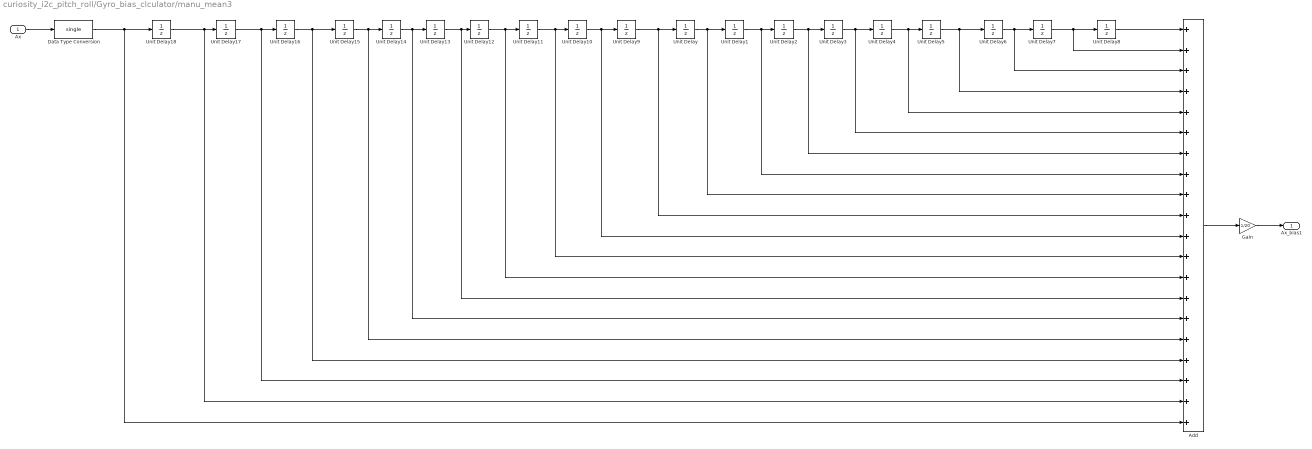
== system curiosity_i2c_pitch_roll/Gyro_bias_clculator/manu_mean3 ==
  Ax : Inport
  Add : Sum  Inputs=++++++++++++++++++++
  Data Type Conversion : DataTypeConversion  OutDataTypeStr=single  SaturateOnIntegerOverflow=off  RndMeth=Floor
  Gain : Gain  Gain=1/20
  Unit Delay{,1..18} (19 alike) : UnitDelay  SampleTime=-1  HasFrameUpgradeWarning=on
  Ax_bias1 : Outport
  wires:
  Unit Delay2/1 -> Add/7, Unit Delay3/1
  Unit Delay1/1 -> Add/8, Unit Delay2/1
  Unit Delay/1 -> Add/9, Unit Delay1/1
  Unit Delay7/1 -> Add/2, Unit Delay8/1
  Unit Delay5/1 -> Add/4, Unit Delay6/1
  Unit Delay4/1 -> Add/5, Unit Delay5/1
  Unit Delay3/1 -> Add/6, Unit Delay4/1
  Unit Delay6/1 -> Add/3, Unit Delay7/1
  Data Type Conversion/1 -> Add/20, Unit Delay18/1
  Add/1 -> Gain/1
  Ax/1 -> Data Type Conversion/1
  Unit Delay8/1 -> Add/1
  Gain/1 -> Ax_bias1/1
  Unit Delay9/1 -> Add/10, Unit Delay/1
  Unit Delay10/1 -> Add/11, Unit Delay9/1
  Unit Delay11/1 -> Add/12, Unit Delay10/1
  Unit Delay12/1 -> Add/13, Unit Delay11/1
  Unit Delay13/1 -> Add/14, Unit Delay12/1
  Unit Delay14/1 -> Add/15, Unit Delay13/1
  Unit Delay15/1 -> Add/16, Unit Delay14/1
  Unit Delay16/1 -> Add/17, Unit Delay15/1
  Unit Delay17/1 -> Add/18, Unit Delay16/1
  Unit Delay18/1 -> Add/19, Unit Delay17/1

== system curiosity_i2c_pitch_roll/MPU9250-AK8963 Accelerometers Gyrometers Magnetometers I2C Interface/Configure MPU-9250 ==
  Enable : EnablePort
  BUS I2C Configure AK8963 mag (MPU-9250) : MCHP_Blockset/BUS I2C/BUS I2C MASTER  I2CRef=2  I2C_IntPriority=5  I2Csequence_txt="Initial-Configuration$     ---     $Start$Write Address:{[0x0C]}    % AK8963 address$Write Data (x1)  Write:{[0x0A]}      % CNTL1$Write Data (x1)  Write:{[0x16]}      % 16bits-100Hz$Stop"  I2Csequence_num=[BFF0000000000000 40E0400000000000 41186A0000000000 41187A2B6F0EC141]$4070000000000000$[3FF0000000000000 40E0400000000000 410065D800000000 410065D9C7810E65]$[4040000000000000 0000000000000000 0000000000000000 4028000000000000]$[4050000000000000 3FF0000000000000 0000000000000000 4024000000000000]$[4050000000000000 3FF0000000000000 0000000000000000 4036000000000000]$[4000000000000000 40E0000000000000 40F86A0000000000 410065D9C7810E65]  InitialConfigurationNum=0  PIN_SDA_TXT=D8 / Pin[58]  PIN_SCL_TXT=D7 / Pin[57]  S_INPUT="[5  5]"  S_OUTPUT=[5]  S_INPUT_Size="[2  2]"  S_OUTPUT_Size=[4]  BlockingMode=off  SequenceCompleted=on  SampleTime=-1  MCHP_MASTERLINK=curiosity_i2c_pitch_roll/CuriosityPlatform Development Board dsPIC33AK128MC106 GP DIM/Microchip Master  MCHP_PORT={I2C 2 Clock}{SCL2}13:0:D7;{I2C 2 SDA}{SDA2}13:0:D8;  ORDERING=0
      settings: SourceProductName=MPLAB Device Blocks for Simulink
  BUS I2C Configure MPU-9250 : MCHP_Blockset/BUS I2C/BUS I2C MASTER  I2CRef=2  I2C_IntPriority=5  I2Csequence_txt="Initial-Configuration$     ---     $Start$Write Address:{MPU_9250.ADDR}    % MPU9250 I2C Address$Write Data (x1)  Write:{[0x6B]}      % ADR PWR_MGMT_1$Write Data (x1)  Write:{[0x01]}      % PWR_MGMT_1$Stop$Start$Write Address:{MPU_9250.ADDR}    % MPU9250 I2C Address$Write Data (x1)  Write:{[0x1A]}      % CONFIG reg addr$Write Data (x1)  Write:{MPU_9250.Config}      % CONFIG$Write Data (x1)  Write:{MPU_9250.Gyro_Config}      % GYRO_CONFIG$Write Data (x1)  Write:{MPU_9250.Accel_Config}      % ACCEL_CONFIG$Write Data (x1)  Write:{MPU_9250.Accel_Config2}      % ACCEL_CONFIG2$Stop"  I2Csequence_num=[BFF0000000000000 40E0400000000000 41186A0000000000 41187A2B6F0EC141]$4070000000000000$[3FF0000000000000 40E0200000000000 40F86A0000000000 40F866E066594CA2]$[4040000000000000 0000000000000000 0000000000000000 FFF8000000000000 4053400000000000 4054000000000000 4055400000000000 4057C00000000000 404C800000000000 4049000000000000 404A800000000000 4048000000000000 4047000000000000 4050400000000000 4051000000000000 4051000000000000 4054800000000000]$[4050000000000000 3FF0000000000000 0000000000000000 405AC00000000000]$[4050000000000000 3FF0000000000000 0000000000000000 3FF0000000000000]$[4000000000000000 40E0000000000000 41186A0000000000 4118666E3C87173F]$[3FF0000000000000 40E0200000000000 40F86A0000000000 40F866E066594CA2]$[4040000000000000 0000000000000000 0000000000000000 FFF8000000000000 4053400000000000 4054000000000000 4055400000000000 4057C00000000000 404C800000000000 4049000000000000 404A800000000000 4048000000000000 4047000000000000 4050400000000000 4051000000000000 4051000000000000 4054800000000000]$[4050000000000000 3FF0000000000000 0000000000000000 403A000000000000]$[4050000000000000 3FF0000000000000 0000000000000000 FFF8000000000000 4053400000000000 4054000000000000 4055400000000000 4057C00000000000 404C800000000000 4049000000000000 404A800000000000 4048000000000000 4047000000000000 4050C00000000000 405BC00000000000 405B800000000000 4059800000000000 405A400000000000 4059C00000000000]$[4050000000000000 3FF0000000000000 0000000000000000 FFF8000000000000 4053400000000000 4054000000000000 4055400000000000 4057C00000000000 404C800000000000 4049000000000000 404A800000000000 4048000000000000 4047000000000000 4051C00000000000 405E400000000000 405C800000000000 405BC00000000000 4057C00000000000 4050C00000000000 405BC00000000000 405B800000000000 4059800000000000 405A400000000000 4059C00000000000]$[4050000000000000 3FF0000000000000 0000000000000000 FFF8000000000000 4053400000000000 4054000000000000 4055400000000000 4057C00000000000 404C800000000000 4049000000000000 404A800000000000 4048000000000000 4047000000000000 4050400000000000 4058C00000000000 4058C00000000000 4059400000000000 405B000000000000 4057C00000000000 4050C00000000000 405BC00000000000 405B800000000000 4059800000000000 405A400000000000 4059C00000000000]$[4050000000000000 3FF0000000000000 0000000000000000 FFF8000000000000 4053400000000000 4054000000000000 4055400000000000 4057C00000000000 404C800000000000 4049000000000000 404A800000000000 4048000000000000 4047000000000000 4050400000000000 4058C00000000000 4058C00000000000 4059400000000000 405B000000000000 4057C00000000000 4050C00000000000 405BC00000000000 405B800000000000 4059800000000000 405A400000000000 4059C00000000000 4049000000000000]$[4000000000000000 40E0000000000000 40F86A0000000000 410065D9C7810E65]  InitialConfigurationNum=0  PIN_SDA_TXT=D8 / Pin[58]  PIN_SCL_TXT=D7 / Pin[57]  S_INPUT="[5  5]"  S_OUTPUT=[5]  S_INPUT_Size="[2  2]"  S_OUTPUT_Size=[4]  BlockingMode=off  SequenceCompleted=on  SampleTime=-1  MCHP_MASTERLINK=curiosity_i2c_pitch_roll/CuriosityPlatform Development Board dsPIC33AK128MC106 GP DIM/Microchip Master  MCHP_PORT={I2C 2 Clock}{SCL2}13:0:D7;{I2C 2 SDA}{SDA2}13:0:D8;  ORDERING=0
      settings: SourceProductName=MPLAB Device Blocks for Simulink
  Logical Operator : Logic  AllPortsSameDT=off  OutDataTypeStr=boolean
  Ok : Outport  InitialOutput=0  VectorParamsAs1DForOutWhenUnconnected=off
  wires:
  Logical Operator/1 -> Ok/1
  BUS I2C Configure MPU-9250/1 -> Logical Operator/1
  BUS I2C Configure AK8963 mag (MPU-9250)/1 -> Logical Operator/2

== system curiosity_i2c_pitch_roll/MPU9250-AK8963 Accelerometers Gyrometers Magnetometers I2C Interface/MPU-9250 ByPass I2C to AK8963 magnetometer Read IDs ==
  Enable : EnablePort
  MPU-9250 ByPass I2C to AK8963 magnetometer Read IDs : MCHP_Blockset/BUS I2C/BUS I2C MASTER  I2CRef=2  I2C_IntPriority=5  I2Csequence_txt="Initial-Configuration$     ---     $Start$Write Address:{MPU_9250.ADDR}    % MPU9250 I2C Address$Write Data (x1)  Write:{[0x75]}      % Who Am I (0x71)$Re-Start    % Re-Start when not followed with either Read or Write action rethrow Address$Write Address:{MPU_9250.ADDR}    % MPU9250 I2C Address$Read Data (x1)  Read:{ID MPU9250}    % ID= 0x71 (113)$Stop$Start$Write Address:{MPU_9250.ADDR}    % MPU9250 I2C Address$Write Data (x1)  Write:{[0x37]}      % INT_PIN_CFG$Write Data (x1)  Write:{[0x02]}      % I2C Pass_Through toward AK8963$Stop$Start$Write Address:{0x0C}    % AK8963 address$Write Data (x1)  Write:{[0x00]}      % ID$Re-Start$Write Address:{[0x0C]}    % AK8963 address$Read Data (x1)  Read:{ID AK8963}    % ID 0x48 (72)$Stop"  I2Csequence_num=[BFF0000000000000 40E0400000000000 41186A0000000000 41187A2B6F0EC141]$4070000000000000$[3FF0000000000000 40E0200000000000 40F86A0000000000 40F866E066594CA2]$[4040000000000000 0000000000000000 0000000000000000 FFF8000000000000 4053400000000000 4054000000000000 4055400000000000 4057C00000000000 404C800000000000 4049000000000000 404A800000000000 4048000000000000 4047000000000000 4050400000000000 4051000000000000 4051000000000000 4054800000000000]$[4050000000000000 3FF0000000000000 0000000000000000 405D400000000000]$[4008000000000000 40E0000000000000 40F86A0000000000 410065D9C7810E65]$[4040000000000000 0000000000000000 0000000000000000 FFF8000000000000 4053400000000000 4054000000000000 4055400000000000 4057C00000000000 404C800000000000 4049000000000000 404A800000000000 4048000000000000 4047000000000000 4050400000000000 4051000000000000 4051000000000000 4054800000000000]$[4060000000000000 3FF0000000000000]$[4000000000000000 40E0000000000000 40F86A0000000000 410065D9C7810E65]$[3FF0000000000000 40E0200000000000 40F86A0000000000 40F866E066594CA2]$[4040000000000000 0000000000000000 0000000000000000 FFF8000000000000 4053400000000000 4054000000000000 4055400000000000 4057C00000000000 404C800000000000 4049000000000000 404A800000000000 4048000000000000 4047000000000000 4050400000000000 4051000000000000 4051000000000000 4054800000000000]$[4050000000000000 3FF0000000000000 0000000000000000 404B800000000000]$[4050000000000000 3FF0000000000000 0000000000000000 4000000000000000]$[4000000000000000 40E0000000000000 40F86A0000000000 410065D9C7810E65]$[3FF0000000000000 40E0400000000000 410065D800000000 410065D9C7810E65]$[4040000000000000 0000000000000000 0000000000000000 4028000000000000]$[4050000000000000 3FF0000000000000 0000000000000000 0000000000000000]$[4008000000000000 40E0400000000000 410065D800000000 410065D9C7810E65]$[4040000000000000 0000000000000000 0000000000000000 4028000000000000]$[4060000000000000 3FF0000000000000]$[4000000000000000 40E0000000000000 40F86A0000000000 410065D9C7810E65]  InitialConfigurationNum=0  PIN_SDA_TXT=D8 / Pin[58]  PIN_SCL_TXT=D7 / Pin[57]  S_INPUT="[5  5]"  S_OUTPUT=[5]  S_INPUT_Size="[2  2]"  S_OUTPUT_Size=[4]  BlockingMode=off  SequenceCompleted=on  SampleTime=[0.1]  MCHP_MASTERLINK=curiosity_i2c_pitch_roll/CuriosityPlatform Development Board dsPIC33AK128MC106 GP DIM/Microchip Master  MCHP_PORT={I2C 2 Clock}{SCL2}13:0:D7;{I2C 2 SDA}{SDA2}13:0:D8;  ORDERING=0
      settings: SourceProductName=MPLAB Device Blocks for Simulink
  Ok : Outport  InitialOutput=0  VectorParamsAs1DForOutWhenUnconnected=off
  Id MPU9250 : Outport  Port=2  VectorParamsAs1DForOutWhenUnconnected=off
  "Id AK8963 " : Outport  Port=3  VectorParamsAs1DForOutWhenUnconnected=off
  wires:
  MPU-9250 ByPass I2C to AK8963 magnetometer Read IDs/1 -> Ok/1
  MPU-9250 ByPass I2C to AK8963 magnetometer Read IDs/2 -> Id MPU9250/1
  MPU-9250 ByPass I2C to AK8963 magnetometer Read IDs/3 -> "Id AK8963 "/1

== system curiosity_i2c_pitch_roll/MPU9250-AK8963 Accelerometers Gyrometers Magnetometers I2C Interface/Sample magnetometers on MPU-9250-AK8963 ==
  Enable : EnablePort
  BUS I2C Read Magnetometers @ 100Hz : MCHP_Blockset/BUS I2C/BUS I2C MASTER  I2CRef=2  I2C_IntPriority=5  I2Csequence_txt="Initial-Configuration$     ---     $Start$Write Address:{[0x0C]}    % AK8963 address$Write Data (x1)  Write:{[0x02]}      % Addr Start readding$Re-Start$Write Address:{[0x0C]}    % AK8963 address$Read Data (x1)  Read:{ST1}    % ST1$Read Data (x2)  Read:{MAG-X}    % MAG$Read Data (x2)  Read:{MAG-Y}    % MAG$Read Data (x2)  Read:{MAG-Z}    % MAG$Read Data (x1)  Read:{ST2}    % ST2 read required$Stop"  I2Csequence_num=[BFF0000000000000 40E0400000000000 41186A0000000000 41187A2B6F0EC141]$4070000000000000$[3FF0000000000000 40E0400000000000 410065D800000000 410065D9C7810E65]$[4040000000000000 0000000000000000 0000000000000000 4028000000000000]$[4050000000000000 3FF0000000000000 0000000000000000 4000000000000000]$[4008000000000000 40E0400000000000 410065D800000000 410065D9C7810E65]$[4040000000000000 0000000000000000 0000000000000000 4028000000000000]$[4060000000000000 3FF0000000000000]$[4060000000000000 4000000000000000]$[4060000000000000 4000000000000000]$[4060000000000000 4000000000000000]$[4060000000000000 3FF0000000000000]$[4000000000000000 40E0000000000000 40F86A0000000000 410065D9C7810E65]  InitialConfigurationNum=0  PIN_SDA_TXT=D8 / Pin[58]  PIN_SCL_TXT=D7 / Pin[57]  S_INPUT="[5  5]"  S_OUTPUT=[5]  S_INPUT_Size="[2  2]"  S_OUTPUT_Size=[4]  BlockingMode=off  SequenceCompleted=on  SampleTime=-1  MCHP_MASTERLINK=curiosity_i2c_pitch_roll/CuriosityPlatform Development Board dsPIC33AK128MC106 GP DIM/Microchip Master  MCHP_PORT={I2C 2 Clock}{SCL2}13:0:D7;{I2C 2 SDA}{SDA2}13:0:D8;  ORDERING=0
      settings: SourceProductName=MPLAB Device Blocks for Simulink
  Concat7 : Subsystem
  Concat8 : Subsystem
  Concat9 : Subsystem
  Ok : Outport  InitialOutput=0  VectorParamsAs1DForOutWhenUnconnected=off
  ST1 : Outport  Port=2  VectorParamsAs1DForOutWhenUnconnected=off
  MAG-X : Outport  Port=3  VectorParamsAs1DForOutWhenUnconnected=off
  MAX-Y : Outport  Port=4  VectorParamsAs1DForOutWhenUnconnected=off
  MAG-Z : Outport  Port=5  VectorParamsAs1DForOutWhenUnconnected=off
  ST2 : Outport  Port=6  VectorParamsAs1DForOutWhenUnconnected=off
  wires:
  BUS I2C Read Magnetometers @ 100Hz/6 -> ST2/1
  BUS I2C Read Magnetometers @ 100Hz/5 -> Concat9/1("[L H]")
  BUS I2C Read Magnetometers @ 100Hz/4 -> Concat8/1("[L H]")
  BUS I2C Read Magnetometers @ 100Hz/3 -> Concat7/1("[L H]")
  BUS I2C Read Magnetometers @ 100Hz/2 -> ST1/1
  BUS I2C Read Magnetometers @ 100Hz/1 -> Ok/1
  Concat7/1(HL) -> MAG-X/1  "U1 CH7"
  Concat9/1(HL) -> MAG-Z/1  "U1 CH9"
  Concat8/1(HL) -> MAX-Y/1  "U1 CH8"
